simulink model "orbit_propagation"  (R2023a)
settings: Solver=VariableStepAuto  StartTime=0.0  StopTime=10.0  RelTol=1e-3
model workspace (MATLAB code in the model file):
  | %--------------------------------------------------------------------------
  | %
  | % IERS: Management of IERS time and polar motion data
  | %
  | % Last modified:   2018/02/01   M. Mahooti
  | %
  | %--------------------------------------------------------------------------
  | function [x_pole,y_pole,UT1_UTC,LOD,dpsi,deps,dx_pole,dy_pole,TAI_UTC] = IERS(eop,Mjd_UTC,interp,astro_constants)
  | 
  | if (nargin == 2)
  |    interp = 'n';
  | end
  | 
  | if (interp =='l')
  |     % linear interpolation
  |     mjd = (floor(Mjd_UTC));
  |     i = find(mjd==eop(4,:),1,'first');
  |     preeop = eop(:,i);
  |     nexteop = eop(:,i+1);
  |     mfme = 1440*(Mjd_UTC-floor(Mjd_UTC));
  |     fixf = mfme/1440;
  |     % Setting of IERS Earth rotation parameters
  |     % (UT1-UTC [s], TAI-UTC [s], x ["], y ["])
  |     x_pole  = preeop(5)+(nexteop(5)-preeop(5))*fixf;
  |     y_pole  = preeop(6)+(nexteop(6)-preeop(6))*fixf;
  | 	UT1_UTC = preeop(7)+(nexteop(7)-preeop(7))*fixf;
  |     LOD     = preeop(8)+(nexteop(8)-preeop(8))*fixf;
  |     dpsi    = preeop(9)+(nexteop(9)-preeop(9))*fixf;
  |     deps    = preeop(10)+(nexteop(10)-preeop(10))*fixf;
  |     dx_pole = preeop(11)+(nexteop(11)-preeop(11))*fixf;
  |     dy_pole = preeop(12)+(nexteop(12)-preeop(12))*fixf;
  |     TAI_UTC = preeop(13);
  | 
  |     x_pole  = x_pole/astro_constants.Arcs;  % Pole coordinate [rad]
  |     y_pole  = y_pole/astro_constants.Arcs;  % Pole coordinate [rad]
  |     dpsi    = dpsi/astro_constants.Arcs;
  |     deps    = deps/astro_constants.Arcs;
  |     dx_pole = dx_pole/astro_constants.Arcs; % Pole coordinate [rad]
  |     dy_pole = dy_pole/astro_constants.Arcs; % Pole coordinate [rad]
  | elseif (interp =='n')
  |     mjd = (floor(Mjd_UTC));
  |     i = find(mjd==eop(4,:),1,'first');
  |     eop = eop(:,i);
  |     % Setting of IERS Earth rotation parameters
  |     % (UT1-UTC [s], TAI-UTC [s], x ["], y ["])
  |     x_pole  = eop(5)/astro_constants.Arcs;  % Pole coordinate [rad]
  |     y_pole  = eop(6)/astro_constants.Arcs;  % Pole coordinate [rad]
  | 	UT1_UTC = eop(7);             % UT1-UTC time difference [s]
  |     LOD     = eop(8);             % Length of day [s]
  |     dpsi    = eop(9)/astro_constants.Arcs;
  |     deps    = eop(10)/astro_constants.Arcs;
  |     dx_pole = eop(11)/astro_constants.Arcs; % Pole coordinate [rad]
  |     dy_pole = eop(12)/astro_constants.Arcs; % Pole coordinate [rad]
  | 	TAI_UTC = eop(13);            % TAI-UTC time difference [s]
  | end
values from neighbouring files (symbols this model uses):
  astro_constants = 6.2831853071795862    [constants.sldd]
  eopdata = 1962.0 1.0 1.0 37665.0 -0.0127 0.213 0.0326338 0.001723 0.064261 0.006067 0.0 0.0 2.0 1962.0 1.0 2.0 37666.0 -0.0159 0.2141 0.0320547 0.001669 0.063979 0.00629 0.0 0.0 2.0 1962.0 1.0 3.0 37667.0 -0.019 0.2152 0.0315526 0.001582 0.06387 0.006515 0.0 0.0 2.0 1962.0 1.0 4.0 37668.0 -0.021999 0.216301 0.0311435 0.001496 0.063893 0.006574 0.0 0.0 2.0 1962.0 1.0 5.0 37669.0 -0.024799 0.217301 0.0308154    [constants.sldd]
undefined symbols (not defined in the file or in its folder): km, m, s
libraries: aerolibconvert2 x2, aerolibatmos2 x1
settings Model: DataDictionary=constants.sldd  Creator=orous  LastModifiedBy=orous

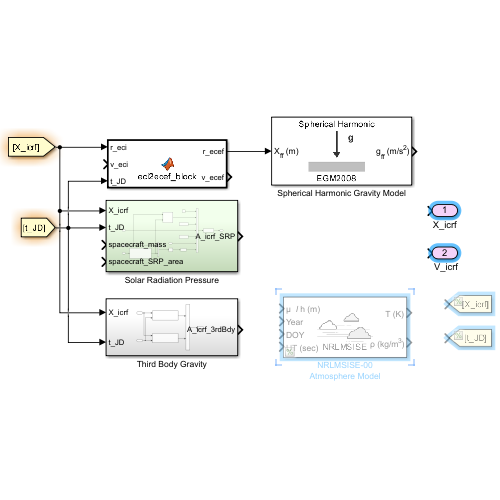
[thumbnail: Simulink's stored preview of the top-level diagram]
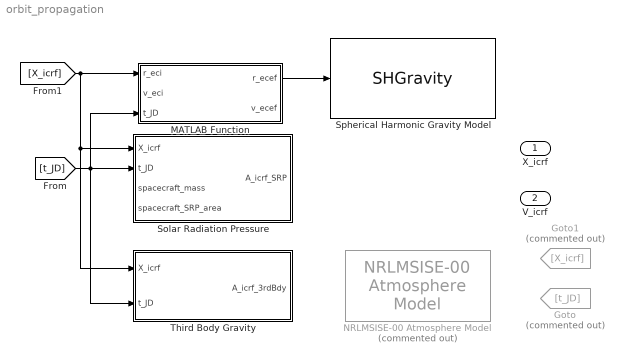
== system orbit_propagation ==
  Goto : Goto  Commented=on  GotoTag=t_JD
  Goto1 : Goto  Commented=on  GotoTag=X_icrf
  MATLAB Function : MATLAB Function  TreatAsAtomicUnit=on
  NRLMSISE-00 Atmosphere Model : aerolibatmos2/NRLMSISE-00 Atmosphere Model  Commented=on  units=Metric (MKS)  lst_input=off  flux_ap_input=off  flags_input=Internal  flags=ones(1,23)  oxygen_in=on  action=Warning
  Solar Radiation Pressure : Subsystem
  Spherical Harmonic Gravity Model : SHGravity
  Third Body Gravity : Subsystem
  X_icrf : Outport
  " V_icrf" : Outport  Port=2
  wires:
  [X_icrf] -> Third Body Gravity/1(X_icrf), Solar Radiation Pressure/1(X_icrf), MATLAB Function/1(r_eci)
  MATLAB Function/1(r_ecef) -> Spherical Harmonic Gravity Model/1
  [t_JD] -> Third Body Gravity/2(t_JD), MATLAB Function/3(t_JD), Solar Radiation Pressure/2(t_JD)

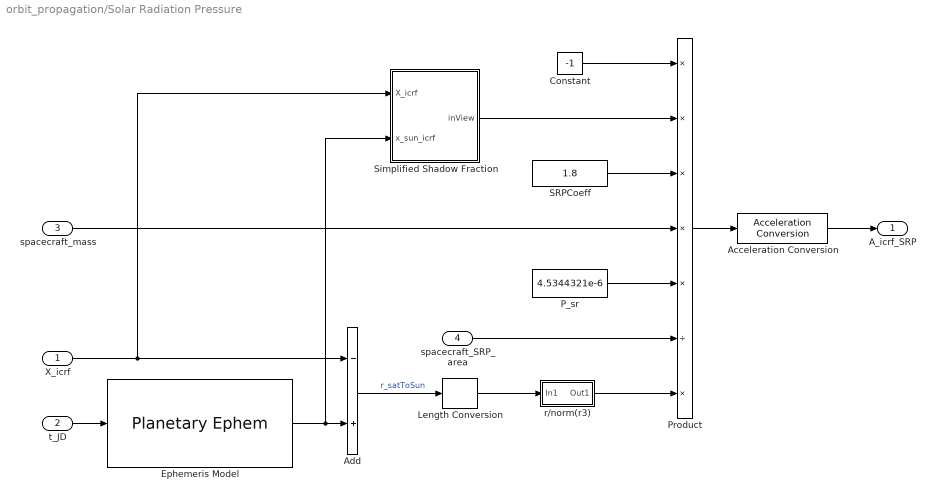
== system orbit_propagation/Solar Radiation Pressure ==
  X_icrf : Inport
  t_JD : Inport  Port=2
  spacecraft_mass : Inport  Port=3
  spacecraft_SRP_area : Inport  Port=4
  Acceleration Conversion : aerolibconvert2/Acceleration Conversion  IU=m/s^2  OU=km/s^2
  Add : Sum  Inputs=-+
  Constant : Constant  Value=-1
  Ephemeris Model : PlanetaryEphem  target=Sun  outputVelocity=off
      settings: AttributesFormatString=|
      | %<nCenter> to %<nTarget>
      | JPL Model: %<de>
  Length Conversion : aerolibconvert2/Length Conversion  IU=km  OU=m
  P_sr : Constant  Value=4.5344321e-6
  Product : Product  Inputs=*****/*
  SRPCoeff : Constant  Value=1.8
  Simplified Shadow Fraction : Subsystem
  r/norm(r3) : Subsystem
  A_icrf_SRP : Outport
  wires:
  SRPCoeff/1 -> Product/3
  P_sr/1 -> Product/5
  t_JD/1 -> Ephemeris Model/1
  X_icrf/1 -> Simplified Shadow Fraction/1(X_icrf), Add/1
  Add/1 -> Length Conversion/1  "r_satToSun"
  Ephemeris Model/1 -> Simplified Shadow Fraction/2(x_sun_icrf), Add/2
  r/norm(r3)/1(Out1) -> Product/7
  Constant/1 -> Product/1
  Simplified Shadow Fraction/1(inView) -> Product/2
  Product/1 -> Acceleration Conversion/1
  Length Conversion/1 -> r/norm(r3)/1(In1)
  Acceleration Conversion/1 -> A_icrf_SRP/1
  spacecraft_mass/1 -> Product/4
  spacecraft_SRP_area/1 -> Product/6

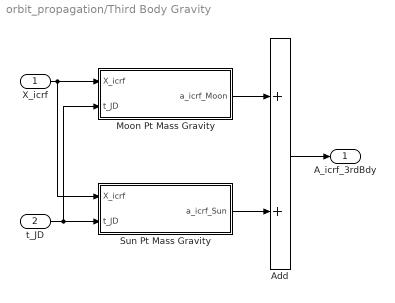
== system orbit_propagation/Third Body Gravity ==
  X_icrf : Inport
  t_JD : Inport  Port=2
  Add : Sum  Inputs=2
  Moon Pt Mass Gravity : Subsystem
  Sun Pt Mass Gravity : Subsystem
  A_icrf_3rdBdy : Outport
  wires:
  Sun Pt Mass Gravity/1(a_icrf_Sun) -> Add/2
  Moon Pt Mass Gravity/1(a_icrf_Moon) -> Add/1
  X_icrf/1 -> Moon Pt Mass Gravity/1(X_icrf), Sun Pt Mass Gravity/1(X_icrf)
  t_JD/1 -> Moon Pt Mass Gravity/2(t_JD), Sun Pt Mass Gravity/2(t_JD)
  Add/1 -> A_icrf_3rdBdy/1

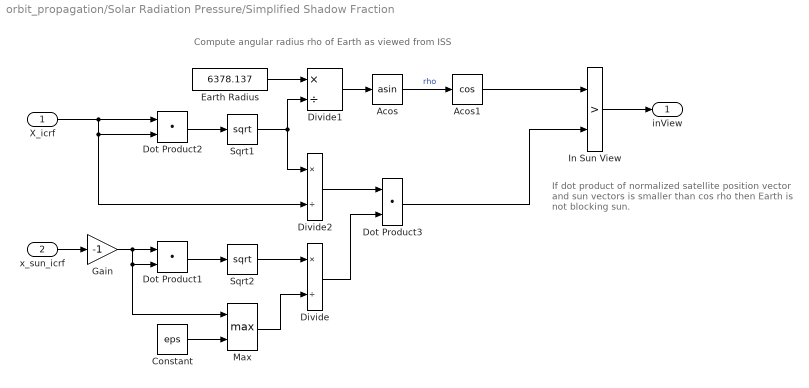
== system orbit_propagation/Solar Radiation Pressure/Simplified Shadow Fraction ==
  note: Compute angular radius rho of Earth as viewed from ISS
  note: If dot product of normalized satellite position vector and sun vectors is smaller than cos rho then Earth is not blocking sun.
  X_icrf : Inport
  x_sun_icrf : Inport  Port=2  SampleTime=0
  Acos : Trigonometry  Operator=asin
  Acos1 : Trigonometry  Operator=cos
  Constant : Constant  Value=eps
  Divide : Product  Inputs=*/
  Divide1 : Product  Inputs=*/
  Divide2 : Product  Inputs=*/
  Dot Product1 : DotProduct  OutDataTypeStr=Inherit: Inherit via internal rule
  Dot Product2 : DotProduct  OutDataTypeStr=Inherit: Inherit via internal rule
  Dot Product3 : DotProduct  OutDataTypeStr=Inherit: Inherit via internal rule
  Earth Radius : Constant  Value=6378.137  VectorParams1D=off  SampleTime=0
  Gain : Gain  Gain=-1
  In Sun View : RelationalOperator  Operator=>  OutDataTypeStr=boolean  ZeroCross=off  RndMeth=Simplest  InputSameDT=off
  Max : MinMax  Function=max  Inputs=2
  Sqrt1 : Sqrt
  Sqrt2 : Sqrt
  inView : Outport  SampleTime=0
  wires:
  Gain/1 -> Max/1, Dot Product1/2, Dot Product1/1
  In Sun View/1 -> inView/1
  X_icrf/1 -> Divide2/2, Dot Product2/2, Dot Product2/1
  Earth Radius/1 -> Divide1/1
  Dot Product2/1 -> Sqrt1/1
  x_sun_icrf/1 -> Gain/1
  Sqrt1/1 -> Divide2/1, Divide1/2
  Divide1/1 -> Acos/1
  Acos/1 -> Acos1/1  "rho"
  Divide/1 -> Dot Product3/2
  Acos1/1 -> In Sun View/1
  Divide2/1 -> Dot Product3/1
  Dot Product3/1 -> In Sun View/2
  Sqrt2/1 -> Divide/1
  Dot Product1/1 -> Sqrt2/1
  Constant/1 -> Max/2
  Max/1 -> Divide/2

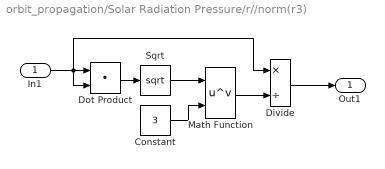
== system orbit_propagation/Solar Radiation Pressure/r//norm(r3) ==
  In1 : Inport
  Constant : Constant  Value=3
  Divide : Product  Inputs=*/
  Dot Product : DotProduct  OutDataTypeStr=Inherit: Inherit via internal rule
  Math Function : Math  Operator=pow
  Sqrt : Sqrt
  Out1 : Outport
  wires:
  Math Function/1 -> Divide/2
  Constant/1 -> Math Function/2
  In1/1 -> Divide/1, Dot Product/2, Dot Product/1
  Sqrt/1 -> Math Function/1
  Dot Product/1 -> Sqrt/1
  Divide/1 -> Out1/1

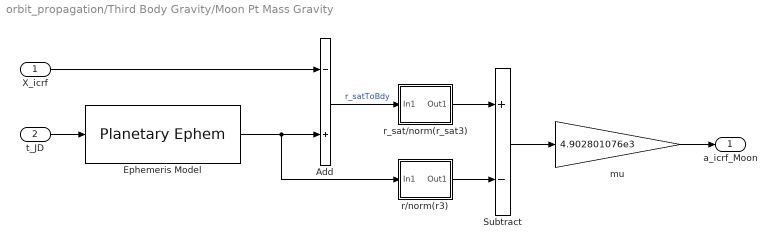
== system orbit_propagation/Third Body Gravity/Moon Pt Mass Gravity ==
  X_icrf : Inport
  t_JD : Inport  Port=2
  Add : Sum  Inputs=-+
  Ephemeris Model : PlanetaryEphem  outputVelocity=off
      settings: AttributesFormatString=|
      | %<nCenter> to %<nTarget>
      | JPL Model: %<de>
  Subtract : Sum  Inputs=+-
  mu : Gain  Gain=4.902801076e3
  r/norm(r3) : Subsystem
  r_sat/norm(r_sat3) : Subsystem
  a_icrf_Moon : Outport
  wires:
  mu/1 -> a_icrf_Moon/1
  r_sat/norm(r_sat3)/1(Out1) -> Subtract/1
  Subtract/1 -> mu/1
  Ephemeris Model/1 -> Add/2, r/norm(r3)/1(In1)
  X_icrf/1 -> Add/1
  Add/1 -> r_sat/norm(r_sat3)/1(In1)  "r_satToBdy"
  r/norm(r3)/1(Out1) -> Subtract/2
  t_JD/1 -> Ephemeris Model/1

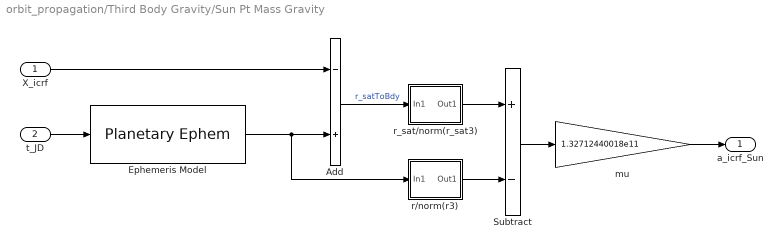
== system orbit_propagation/Third Body Gravity/Sun Pt Mass Gravity ==
  X_icrf : Inport
  t_JD : Inport  Port=2
  Add : Sum  Inputs=-+
  Ephemeris Model : PlanetaryEphem  target=Sun  outputVelocity=off
      settings: AttributesFormatString=|
      | %<nCenter> to %<nTarget>
      | JPL Model: %<de>
  Subtract : Sum  Inputs=+-
  mu : Gain  Gain=1.32712440018e11
  r/norm(r3) : Subsystem
  r_sat/norm(r_sat3) : Subsystem
  a_icrf_Sun : Outport
  wires:
  t_JD/1 -> Ephemeris Model/1
  r/norm(r3)/1(Out1) -> Subtract/2
  Add/1 -> r_sat/norm(r_sat3)/1(In1)  "r_satToBdy"
  X_icrf/1 -> Add/1
  Ephemeris Model/1 -> r/norm(r3)/1(In1), Add/2
  Subtract/1 -> mu/1
  r_sat/norm(r_sat3)/1(Out1) -> Subtract/1
  mu/1 -> a_icrf_Sun/1

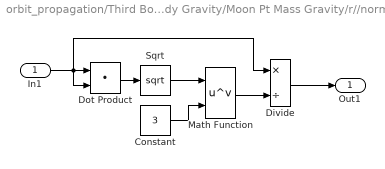
== system orbit_propagation/Third Body Gravity/Moon Pt Mass Gravity/r//norm(r3) ==
  In1 : Inport
  Constant : Constant  Value=3
  Divide : Product  Inputs=*/
  Dot Product : DotProduct  OutDataTypeStr=Inherit: Inherit via internal rule
  Math Function : Math  Operator=pow
  Sqrt : Sqrt
  Out1 : Outport
  wires:
  Math Function/1 -> Divide/2
  Constant/1 -> Math Function/2
  In1/1 -> Divide/1, Dot Product/2, Dot Product/1
  Sqrt/1 -> Math Function/1
  Dot Product/1 -> Sqrt/1
  Divide/1 -> Out1/1

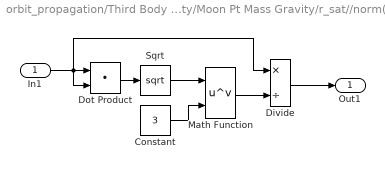
== system orbit_propagation/Third Body Gravity/Moon Pt Mass Gravity/r_sat//norm(r_sat3) ==
  In1 : Inport
  Constant : Constant  Value=3
  Divide : Product  Inputs=*/
  Dot Product : DotProduct  OutDataTypeStr=Inherit: Inherit via internal rule
  Math Function : Math  Operator=pow
  Sqrt : Sqrt
  Out1 : Outport
  wires:
  Divide/1 -> Out1/1
  Dot Product/1 -> Sqrt/1
  Sqrt/1 -> Math Function/1
  In1/1 -> Dot Product/1, Dot Product/2, Divide/1
  Constant/1 -> Math Function/2
  Math Function/1 -> Divide/2

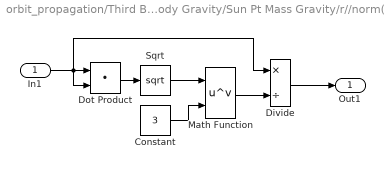
== system orbit_propagation/Third Body Gravity/Sun Pt Mass Gravity/r//norm(r3) ==
  In1 : Inport
  Constant : Constant  Value=3
  Divide : Product  Inputs=*/
  Dot Product : DotProduct  OutDataTypeStr=Inherit: Inherit via internal rule
  Math Function : Math  Operator=pow
  Sqrt : Sqrt
  Out1 : Outport
  wires:
  Divide/1 -> Out1/1
  Dot Product/1 -> Sqrt/1
  Sqrt/1 -> Math Function/1
  In1/1 -> Dot Product/1, Dot Product/2, Divide/1
  Constant/1 -> Math Function/2
  Math Function/1 -> Divide/2

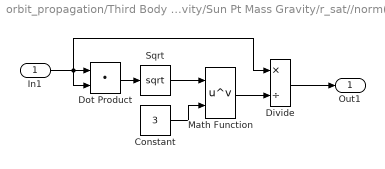
== system orbit_propagation/Third Body Gravity/Sun Pt Mass Gravity/r_sat//norm(r_sat3) ==
  In1 : Inport
  Constant : Constant  Value=3
  Divide : Product  Inputs=*/
  Dot Product : DotProduct  OutDataTypeStr=Inherit: Inherit via internal rule
  Math Function : Math  Operator=pow
  Sqrt : Sqrt
  Out1 : Outport
  wires:
  Math Function/1 -> Divide/2
  Constant/1 -> Math Function/2
  In1/1 -> Divide/1, Dot Product/2, Dot Product/1
  Sqrt/1 -> Math Function/1
  Dot Product/1 -> Sqrt/1
  Divide/1 -> Out1/1

== matlab function orbit_propagation/MATLAB Function ==
  data: r_eci input; v_eci input; r_ecef output; t_JD input; eopdata parameter; astro_constants parameter; v_ecef output
function [r_ecef, v_ecef] = eci2ecef_block(r_eci, v_eci, t_JD, eopdata, astro_constants)

MJD_UTC = t_JD - 2400000.5;
[x_pole, y_pole, UT1_UTC, LOD, TAI_UTC] = IERS(eopdata, MJD_UTC, astro_constants);
TT_UTC = 32.184 + TAI_UTC;
MJD_UT1 = MJD_UTC + UT1_UTC / 86400;
MJD_TT = MJD_UTC + TT_UTC / 86400;

% Interval between fundamental date J2000.0 and given date (JC).
t = ((astro_constants.DJM0 - astro_constants.DJ00) + MJD_TT) / astro_constants.DJC;

% Form bias-precession-nutation matrix
NPB = iauPnm06a(t, astro_constants);
% Form Earth rotation matrix
Theta = iauRz(iauGst06(astro_constants.DJM0, MJD_UT1, astro_constants.DJM0, MJD_TT, NPB, astro_constants), eye(3));
% Polar motion matrix (TIRS->ITRS, IERS 2003)
Pi = iauPom00(x_pole, y_pole, iauSp00(t, astro_constants));

% ICRS to ITRS transformation matrix and derivative
S = zeros(3);
S(1, 2) = 1;
S(2, 1) = -1; % Derivative of Earth rotation
Omega = astro_constants.omega_Earth - 0.843994809 * 1e-9 * LOD; % IERS
dTheta = Omega * S * Theta; % matrix [1/s]
U = Pi * Theta * NPB; % ICRS to ITRS transformation
dU = Pi * dTheta * NPB; % Derivative [1/s]

% Transformation from ICRS to WGS
r_ecef = U * r_eci;
v_ecef = U * v_eci + dU * r_eci;
